simulink library "Lib_CanCommunication"  (R2019b)
settings: Solver=VariableStepAuto  StartTime=0.0  StopTime=10.0  RelTol=1e-3
PostLoadFcn:
  | , if any(exist('dsrtsu_mdlpostloadfcn', 'file') == [2, 3, 6]), try dsrtsu_mdlpostloadfcn('Execute', bdroot); catch fprintf('Error in PostLoadFcn (dsrtsu_mdlpostloadfcn) for model "%s":\n %s\n', bdroot, lasterr); end, end,
undefined symbols (not defined in the file): Counter, CRC, default_customer_can_bus, default_vehicle_state_bus, LateralAcceleration, LongitudinalAcceleration, Motion, Powertrain_1, Steering, steering_angle_range_rad_to_steering_wheel_angle_range_deg_gain, SteeringWheelAngle, SteeringWheelAngleSign, SteeringWheelSpeed, SteeringWheelSpeedSign, SteeringWheelTorque, SteeringWheelTorqueSign, VehicleVelocity, YawRate, YawRateSign
libraries: rtican x8, simulink x6
(part 3 of 3)

== matlab function Lib_CanCommunication/CanCommunication/CustomerCAN/AccInterface/AccelerationInterface/Acceleration_CRC_Calculator ==
  data: counter input; byte0 output; clearanceAI input; activationRequest input; cancelRequest input; accelerationRequest input; clearanceStopDistance input; stopDistanceRequest input; acousticDriverHint input
function byte0 = fcn(counter, clearanceAI, activationRequest, cancelRequest, accelerationRequest, clearanceStopDistance, stopDistanceRequest, acousticDriverHint)

byte0 = Acceleration_CRC_Calculator(counter, clearanceAI, activationRequest, cancelRequest, accelerationRequest, clearanceStopDistance, stopDistanceRequest, acousticDriverHint);

== matlab function Lib_CanCommunication/CanCommunication/CustomerCAN/SteeringInterface/SteeringInterface/MATLAB Function ==
  data: counter input; byte0 output; clearance input; activation input; cancel input; angle input; torque input; torquesign input; anglesign input; advanceanglelim input; frequency input uint8 [0..0]
function byte0 = fcn(counter, clearance, activation, cancel, angle, torque, torquesign, anglesign, advanceanglelim, frequency)

byte0 = Steering_CRC_Calculator(counter, clearance, activation, cancel, angle, torque, torquesign, anglesign, advanceanglelim, frequency);
